simulink model "pose_ctrl_R2017a"  (R2017a)
settings: Solver=FixedStepAuto  StartTime=0.0  StopTime=20  FixedStep=0.0005  RelTol=1e-3
InitFcn:
  | Parameter
values from neighbouring files (symbols this model uses):
  alpha = pi/180 * 13.6    (= 0.237364778271)    [IdealParameter.m]    (also in ParLuk11.m = deg2rad(13.6); Parameter.m = [-alpha_i;alpha_i;-alpha_i;alpha_i;-alpha_i;alpha_i]; ParameterIdeal.m = [-alpha_i;alpha_i;-alpha_i;alpha_i;-alpha_i;alpha_i]; ParameterVIVE.m = [alpha_i;-alpha_i;alpha_i;-alpha_i;alpha_i;-alpha_i])
  alpha_0 = alpha    (= 0.237364778271)    [IdealParameter.m]    (also in Parameter.m = alpha; ParameterIdeal.m = alpha*1.01; ParameterVIVE.m = alpha*1.01; ParameterVO.m = alpha*1.01)
  angular_noise = 0    [IdealParameter.m]    (also in Parameter.m = 0.5; ParameterIdeal.m; ParameterVIVE.m; ParameterVO.m)
  b = 1.1e-06    [IdealParameter.m]    (also in ParLuk11.m = 1.14e-07; Parameter.m = 8.944e-07; ParameterIdeal.m; ParameterVIVE.m)
  b_0 = b*1.15    (= 1.265e-06)    [IdealParameter.m]    (also in Parameter.m = 8.944e-07; ParameterIdeal.m; ParameterVIVE.m; ParameterVO.m)
  beta = 0    [IdealParameter.m]    (also in ParLuk11.m; Parameter.m = [beta_i; beta_i; beta_i; beta_i; beta_i; beta_i]; ParameterIdeal.m = [beta_i; beta_i; beta_i; beta_i; beta_i; beta_i]; ParameterVIVE.m = [beta_i; beta_i; beta_i; beta_i; beta_i; beta_i])
  beta_0 = beta    (= 0)    [IdealParameter.m]    (also in Parameter.m = beta; ParameterIdeal.m = beta*0.99; ParameterVIVE.m = beta*0.99; ParameterVO.m = beta*0.99)
  eta = 1    [Controllability.m]    (also in IdealParameter.m = 75; Parameter.m = 2; ParameterIdeal.m = 40; ParameterVIVE.m = 10)
  eta_rot = 50    [IdealParameter.m]    (also in Parameter.m = 2; ParameterIdeal.m = 20; ParameterVIVE.m = 5; ParameterVO.m = 2)
  g = 9.81    [IdealParameter.m]    (also in ParLuk11.m; Parameter.m; ParameterIdeal.m; ParameterVIVE.m)
  g_0 = g*0.99    (= 9.7119)    [IdealParameter.m]    (also in Parameter.m = 9.81; ParameterIdeal.m = 9.81; ParameterVIVE.m = 9.81; ParameterVO.m = 9.81)
  IB = [Ixx 0 0; 0 Iyy 0; 0 0 Izz]    [IdealParameter.m]    (also in ParLuk11.m; Parameter.m; ParameterIdeal.m; ParameterVIVE.m)
  IB_0 = IB*1.07    [IdealParameter.m]    (also in Parameter.m = IB; ParameterIdeal.m; ParameterVIVE.m; ParameterVO.m)
  k = 5.6e-05    [IdealParameter.m]    (also in ParLuk11.m = 2.98e-06; Parameter.m = 4.472e-05; ParameterIdeal.m; ParameterVIVE.m = 5.13e-05)
  K_0 = Ts/(T_rotor_0+Ts)    (= 0.0384615384615)    [IdealParameter.m]    (also in Parameter.m = 0.230769230769; ParameterIdeal.m; ParameterVIVE.m = 0.0350877192982; ParameterVO.m = 0.214285714286)
  k_0 = k*1.16    (= 6.496e-05)    [IdealParameter.m]    (also in Parameter.m = 4.472e-05; ParameterIdeal.m; ParameterVIVE.m = 5.9508e-05; ParameterVO.m)
  K_P_1 = 15*eye(3)    [IdealParameter.m]    (also in Parameter.m = 2*eye(3); ParameterIdeal.m; ParameterVIVE.m = 10*eye(3); ParameterVO.m = 2*eye(3))
  K_P_2 = 50*eye(3)    [IdealParameter.m]    (also in Parameter.m = 4*eye(3); ParameterIdeal.m; ParameterVIVE.m = 10*eye(3); ParameterVO.m = 4*eye(3))
  K_P_3 = 60*eye(3)    [IdealParameter.m]    (also in Parameter.m = 6*eye(3); ParameterIdeal.m; ParameterVIVE.m = 10*eye(3); ParameterVO.m = 6*eye(3))
  K_P_D = 30*eye(3)    [IdealParameter.m]    (also in ParLuk11.m = 10*eye(3); Parameter.m = 5*eye(3); ParameterIdeal.m; ParameterVIVE.m = 15*eye(3))
  K_P_I = 100*eye(3)    [IdealParameter.m]    (also in ParLuk11.m = 10*eye(3); Parameter.m = 10*eye(3); ParameterIdeal.m = 80*eye(3); ParameterVIVE.m)
  K_P_P = 100*eye(3)    [IdealParameter.m]    (also in ParLuk11.m = 20*eye(3); Parameter.m = 10*eye(3); ParameterIdeal.m = 130*eye(3); ParameterVIVE.m)
  K_R_1 = 40*eye(3)    [IdealParameter.m]    (also in Parameter.m = 2*eye(3); ParameterIdeal.m; ParameterVIVE.m = 10*eye(3); ParameterVO.m = 2*eye(3))
  K_R_2 = 100*eye(3)    [IdealParameter.m]    (also in Parameter.m = 4*eye(3); ParameterIdeal.m; ParameterVIVE.m = 10*eye(3); ParameterVO.m = 4*eye(3))
  K_R_3 = 50*eye(4)    [IdealParameter.m]    (also in Parameter.m = 6*eye(4); ParameterIdeal.m; ParameterVIVE.m = 10*eye(4); ParameterVO.m = 6*eye(4))
  K_R_D = 30*eye(3)    [IdealParameter.m]    (also in ParLuk11.m = 10*eye(3); Parameter.m = 5*eye(3); ParameterIdeal.m; ParameterVIVE.m = 15*eye(3))
  K_R_I = 100*eye(3)    [IdealParameter.m]    (also in ParLuk11.m = 10*eye(3); Parameter.m = 10*eye(3); ParameterIdeal.m = 80*eye(3); ParameterVIVE.m)
  K_R_P = 100*eye(3)    [IdealParameter.m]    (also in ParLuk11.m = 20*eye(3); Parameter.m = 10*eye(3); ParameterIdeal.m = 130*eye(3); ParameterVIVE.m)
  L = 0.4    [IdealParameter.m]    (also in ParLuk11.m = 1; Parameter.m; ParameterIdeal.m; ParameterVIVE.m = 0.6)
  L_0 = L*1.02    (= 0.408)    [IdealParameter.m]    (also in Parameter.m = 0.4; ParameterIdeal.m; ParameterVIVE.m = 0.612; ParameterVO.m)
  lambda = 10    [IdealParameter.m]    (also in Parameter.m = 3; ParameterIdeal.m = 5; ParameterVIVE.m = 5; ParameterVO.m = 3)
  lambda_rot = 10    [IdealParameter.m]    (also in Parameter.m = 3; ParameterIdeal.m; ParameterVIVE.m = 5; ParameterVO.m = 3)
  M = 50    [IdealParameter.m]    (also in Parameter.m = 6; ParameterIdeal.m = 100; ParameterVIVE.m = 5; ParameterVO.m = 6)
  m = 1    [Controllability.m]    (also in IdealParameter.m = 2.5; ParLuk11.m = 0.6; Parameter.m = 4.85; ParameterIdeal.m = 4.85)
  m_0 = m*1.03    (= 2.575)    [IdealParameter.m]    (also in Parameter.m = 4.85; ParameterIdeal.m = 4.9955; ParameterVIVE.m = 4.52994; ParameterVO.m = 4.9955)
  M_rot = 50    [IdealParameter.m]    (also in Parameter.m = 6; ParameterIdeal.m = 15; ParameterVIVE.m = 1; ParameterVO.m = 6)
  omega_noise = 0    [IdealParameter.m]    (also in Parameter.m = sqrt(2)*angular_noise/Ts * pi/180; ParameterIdeal.m; ParameterVIVE.m; ParameterVO.m)
  p_noise = 0    [IdealParameter.m]    (also in Parameter.m = 0.001; ParameterIdeal.m; ParameterVIVE.m; ParameterVO.m)
  T_delay = 0    [IdealParameter.m]    (also in Parameter.m = 0.1; ParameterIdeal.m; ParameterVIVE.m = 0.04; ParameterVO.m = 0.1)
  T_rotor = 0.1    [IdealParameter.m]    (also in Parameter.m; ParameterIdeal.m; ParameterVIVE.m; ParameterVO.m)
  Ts = 1/250    (= 0.004)    [IdealParameter.m]    (also in Parameter.m = 0.03; ParameterIdeal.m; ParameterVIVE.m; ParameterVO.m = 0.03)
  v_noise = 0    [IdealParameter.m]    (also in Parameter.m = sqrt(2)*p_noise/Ts; ParameterIdeal.m; ParameterVIVE.m; ParameterVO.m)
  z_p_0 = T_rotor_0/(T_rotor_0+Ts)    (= 0.961538461538)    [IdealParameter.m]    (also in Parameter.m = 0.769230769231; ParameterIdeal.m; ParameterVIVE.m = 0.964912280702; ParameterVO.m = 0.785714285714)
undefined symbols (not defined in the file or in its folder): DiscIntNeverNeededParam
libraries: simulink x7, vrlib x3, dspmtrx3 x1
(part 1 of 2)
settings Model: Creator=jan  LastModifiedBy=chao

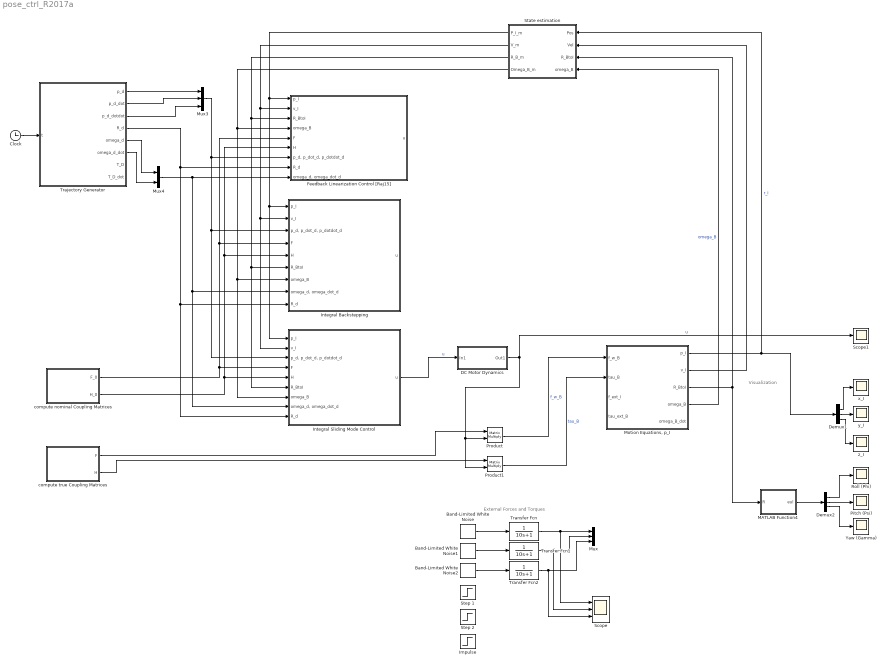
== system pose_ctrl_R2017a ==
  note: External Forces and Torques
  note: Visualization
  Band-Limited White Noise : simulink/Sources/Band-Limited White Noise  Cov=10  Ts=0.1  seed=[28341]  VectorParams1D=off
  Band-Limited White Noise1 : simulink/Sources/Band-Limited White Noise  Cov=10  Ts=0.1  seed=[23342]  VectorParams1D=off
  Band-Limited White Noise2 : simulink/Sources/Band-Limited White Noise  Cov=10  Ts=0.1  seed=[23441]  VectorParams1D=off
  Clock : Clock
  "DC Motor Dynamics " : Subsystem  TreatAsAtomicUnit=on
  Demux1 : Demux  Outputs=3
  Demux2 : Demux  Outputs=3
  Feedback Linearization Control [Raj15] : Subsystem
  Impulse : Step  Time=0.1  Before=[6,0,6]'  After=[0,0,0]'  SampleTime=0  VectorParams1D=off
  Integral Backstepping : Subsystem
  Integral Sliding Mode Control : Subsystem
  MATLAB Function4 : MATLAB Function  TreatAsAtomicUnit=on
  "Motion Equations, p_I" : Subsystem
  Mux : Mux  Inputs=3
  Mux3 : Mux  Inputs=3
  Mux4 : Mux  Inputs=2
  Pitch (Psi) : Scope
  Product : Product  Multiplication=Matrix(*)
  Product1 : Product  Multiplication=Matrix(*)
  Roll (Phi) : Scope
  Scope : Scope  NumInputPorts=3
  Scope1 : Scope
  State estimation : Subsystem
  Step 1 : Step  Before=[0;0;0]  After=[10;1;1]  SampleTime=0  VectorParams1D=off
  Step 2 : Step  Before=[0;0;0]  After=[5;1;1]  SampleTime=0  VectorParams1D=off
  Trajectory Generator : MATLAB Function  TreatAsAtomicUnit=on
  Transfer Fcn : TransferFcn  Denominator=[10 1]
  Transfer Fcn1 : TransferFcn  Denominator=[10 1]
  Transfer Fcn2 : TransferFcn  Denominator=[10 1]
  Yaw (Gamma) : Scope
  compute nominal Coupling Matrices : Subsystem
  compute true Coupling Matrices : Subsystem
  x_I : Scope
  y_I : Scope
  z_I : Scope
  wires:
  Demux2/2 -> Pitch (Psi)/1
  Demux1/3 -> z_I/1
  Demux1/1 -> x_I/1
  "DC Motor Dynamics "/1(Out1) -> Product1/2, Product/2, Scope1/1  "u"
  Demux1/2 -> y_I/1
  Demux2/1 -> Roll (Phi)/1
  compute nominal Coupling Matrices/1(F_0) -> Integral Backstepping/4(F), Feedback Linearization Control [Raj15]/5(F), Integral Sliding Mode Control/4(F)
  Product/1 -> "Motion Equations, p_I"/1("f_w_B ")  "f_w_B"
  compute nominal Coupling Matrices/2("H_0 ") -> Integral Backstepping/5(H), Feedback Linearization Control [Raj15]/6(H), Integral Sliding Mode Control/5(H)
  Product1/1 -> "Motion Equations, p_I"/2(tau_B)  "tau_B"
  Clock/1 -> Trajectory Generator/1(t)
  Trajectory Generator/3(p_d_dotdot) -> Mux3/3
  Trajectory Generator/2(p_d_dot) -> Mux3/2
  Trajectory Generator/1(p_d) -> Mux3/1
  Trajectory Generator/6(omega_d_dot) -> Mux4/2
  Band-Limited White Noise/1 -> Transfer Fcn/1
  Transfer Fcn/1 -> Scope/1, Mux/1
  Transfer Fcn2/1 -> Scope/3, Mux/3
  Band-Limited White Noise1/1 -> Transfer Fcn1/1
  Band-Limited White Noise2/1 -> Transfer Fcn2/1
  Transfer Fcn1/1 -> Scope/2, Mux/2
  Mux3/1 -> Integral Sliding Mode Control/3("p_d, p_dot_d, p_dotdot_d"), Integral Backstepping/3("p_d, p_dot_d, p_dotdot_d"), Feedback Linearization Control [Raj15]/7("p_d, p_dot_d, p_dotdot_d")
  Trajectory Generator/4(R_d) -> Integral Sliding Mode Control/9(R_d), Integral Backstepping/9(R_d), Feedback Linearization Control [Raj15]/8(R_d)
  Trajectory Generator/5(omega_d) -> Mux4/1
  Mux4/1 -> Integral Sliding Mode Control/8("omega_d, omega_dot_d"), Integral Backstepping/8("omega_d, omega_dot_d"), Feedback Linearization Control [Raj15]/9("omega_d, omega_dot_d")
  compute true Coupling Matrices/1(F) -> Product/1
  compute true Coupling Matrices/2(H) -> Product1/1
  "Motion Equations, p_I"/1(p_I) -> Demux1/1, State estimation/1(Pos)  "r_I"
  "Motion Equations, p_I"/3(R_BtoI) -> State estimation/3(R_BtoI), MATLAB Function4/1(R)
  Demux2/3 -> Yaw (Gamma)/1
  MATLAB Function4/1(eul) -> Demux2/1
  Integral Sliding Mode Control/1(u) -> "DC Motor Dynamics "/1(In1)  "u"
  State estimation/3(R_B_m) -> Integral Sliding Mode Control/6(R_BtoI), Integral Backstepping/6(R_BtoI), Feedback Linearization Control [Raj15]/3("R_BtoI ")
  State estimation/2(V_m) -> Integral Sliding Mode Control/2(v_I), Integral Backstepping/2(v_I), Feedback Linearization Control [Raj15]/2(v_I)
  State estimation/1(P_I_m) -> Integral Sliding Mode Control/1(p_I), Integral Backstepping/1(p_I), Feedback Linearization Control [Raj15]/1("p_I ")
  State estimation/4(Omega_B_m) -> Integral Sliding Mode Control/7(omega_B), Integral Backstepping/7(omega_B), Feedback Linearization Control [Raj15]/4(omega_B)
  "Motion Equations, p_I"/2(v_I) -> State estimation/2(Vel)
  "Motion Equations, p_I"/4(omega_B) -> State estimation/4(omega_B)  "omega_B"

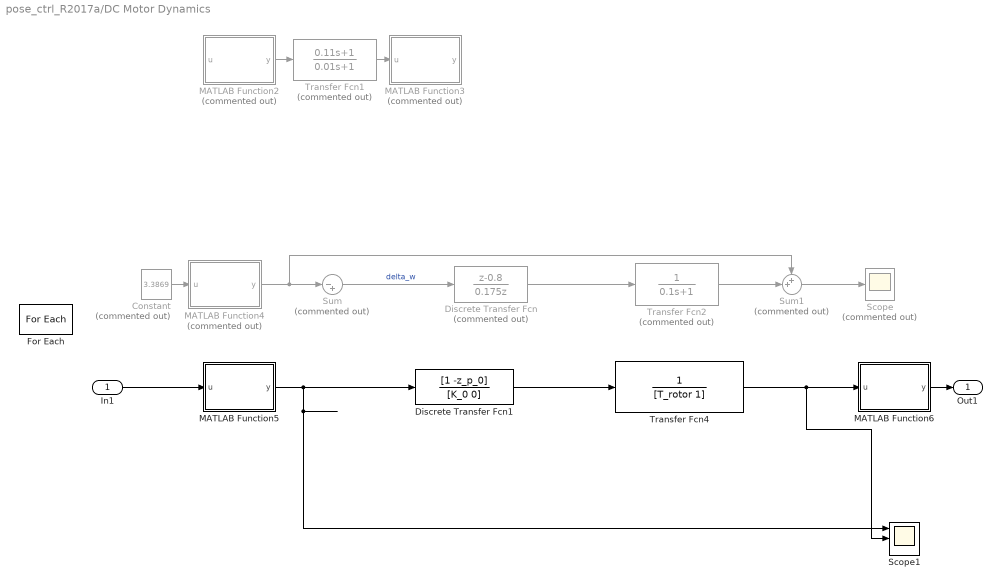
== system pose_ctrl_R2017a/DC Motor Dynamics  ==
  In1 : Inport  Partition=on  PartitionDimension=1  PartitionWidth=1
  Constant : Constant  Commented=on  Value=3.3869
  Discrete Transfer Fcn : DiscreteTransferFcn  Commented=on  Numerator=[1 -0.8]  Denominator=[0.175 0]  SampleTime=Ts
  Discrete Transfer Fcn1 : DiscreteTransferFcn  Numerator=[1 -z_p_0]  Denominator=[K_0 0]  SampleTime=Ts
  For Each : ForEach  DisableCoverage=on  IndexMode=One-based
  MATLAB Function2 : MATLAB Function  Commented=on  TreatAsAtomicUnit=on
  MATLAB Function3 : MATLAB Function  Commented=on  TreatAsAtomicUnit=on
  MATLAB Function4 : MATLAB Function  Commented=on  TreatAsAtomicUnit=on
  MATLAB Function5 : MATLAB Function  TreatAsAtomicUnit=on  SystemSampleTime=Ts
  MATLAB Function6 : MATLAB Function  TreatAsAtomicUnit=on
  Scope : Scope  Commented=on
  Scope1 : Scope  NumInputPorts=3
  Sum : Sum  Commented=on  Inputs=|-+
  Sum1 : Sum  Commented=on  Inputs=++|
  Transfer Fcn1 : TransferFcn  Commented=on  Numerator=[0.11 1]  Denominator=[0.01 1]
  Transfer Fcn2 : TransferFcn  Commented=on  Denominator=[0.1 1]
  Transfer Fcn4 : TransferFcn  Denominator=[T_rotor 1]
  Out1 : Outport  ConcatenationDimension=1
  wires:
  Transfer Fcn1/1 -> MATLAB Function3/1(u)
  MATLAB Function2/1(y) -> Transfer Fcn1/1
  Constant/1 -> MATLAB Function4/1(u)
  MATLAB Function4/1(y) -> Sum1/1, Sum/1
  Sum/1 -> Discrete Transfer Fcn/1  "delta_w"
  In1/1 -> MATLAB Function5/1(u)
  MATLAB Function5/1(y) -> Discrete Transfer Fcn1/1, Scope1/1
  Discrete Transfer Fcn/1 -> Transfer Fcn2/1
  Transfer Fcn2/1 -> Sum1/2
  MATLAB Function6/1(y) -> Out1/1
  Sum1/1 -> Scope/1
  Discrete Transfer Fcn1/1 -> Transfer Fcn4/1
  Transfer Fcn4/1 -> Scope1/2, MATLAB Function6/1(u)

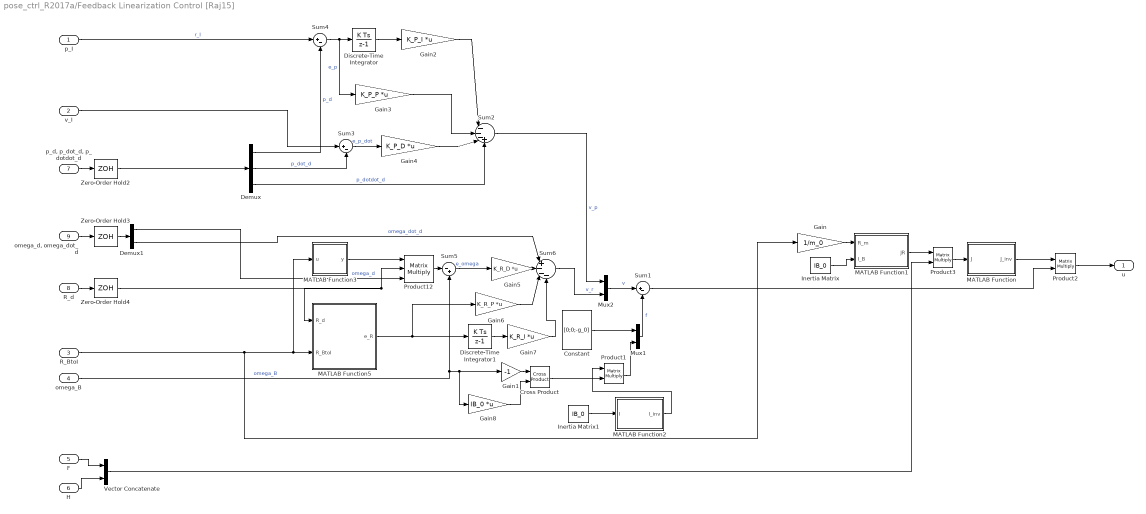
== system pose_ctrl_R2017a/Feedback Linearization Control [Raj15] ==
  "p_I " : Inport
  v_I : Inport  Port=2
  "R_BtoI " : Inport  Port=3
  omega_B : Inport  Port=4
  F : Inport  Port=5
  H : Inport  Port=6
  "p_d, p_dot_d, p_dotdot_d" : Inport  Port=7
  R_d : Inport  Port=8
  "omega_d, omega_dot_d" : Inport  Port=9
  Constant : Constant  Value=[0;0;-g_0]  VectorParams1D=off
  Cross Product : vrlib/Utilities/Cross Product
      settings: SourceProductBaseCode=VR
  Demux : Demux  Outputs=3
  Demux1 : Demux  Outputs=2
  Discrete-Time Integrator : DiscreteIntegrator  InitialCondition=[0;0;0]  InitialConditionSetting=State (most efficient)  SampleTime=Ts  ICPrevOutput=DiscIntNeverNeededParam  ICPrevScaledInput=DiscIntNeverNeededParam
  Discrete-Time Integrator1 : DiscreteIntegrator  InitialCondition=[0;0;0]  InitialConditionSetting=State (most efficient)  SampleTime=Ts  ICPrevOutput=DiscIntNeverNeededParam  ICPrevScaledInput=DiscIntNeverNeededParam
  Gain : Gain  Gain=1/m_0
  Gain1 : Gain  Gain=-1
  Gain2 : Gain  Gain=K_P_I  Multiplication=Matrix(K*u)
  Gain3 : Gain  Gain=K_P_P  Multiplication=Matrix(K*u)
  Gain4 : Gain  Gain=K_P_D  Multiplication=Matrix(K*u)
  Gain5 : Gain  Gain=K_R_D  Multiplication=Matrix(K*u)
  Gain6 : Gain  Gain=K_R_P  Multiplication=Matrix(K*u)
  Gain7 : Gain  Gain=K_R_I  Multiplication=Matrix(K*u)
  Gain8 : Gain  Gain=IB_0  Multiplication=Matrix(K*u)
  Inertia Matrix : Constant  Value=IB_0  VectorParams1D=off
  Inertia Matrix1 : Constant  Value=IB_0  VectorParams1D=off
  MATLAB Function : MATLAB Function  TreatAsAtomicUnit=on
  MATLAB Function1 : MATLAB Function  TreatAsAtomicUnit=on
  MATLAB Function2 : MATLAB Function  TreatAsAtomicUnit=on
  MATLAB Function3 : MATLAB Function  TreatAsAtomicUnit=on
  MATLAB Function5 : MATLAB Function  TreatAsAtomicUnit=on
  Mux1 : Mux  Inputs=2
  Mux2 : Mux  Inputs=2
  Product1 : Product  Multiplication=Matrix(*)
  Product12 : Product  Inputs=***  Multiplication=Matrix(*)
  Product2 : Product  Multiplication=Matrix(*)
  Product3 : Product  Multiplication=Matrix(*)
  Sum1 : Sum  Inputs=|+-
  Sum2 : Sum  Inputs=|---+
  Sum3 : Sum  Inputs=|+-
  Sum4 : Sum  Inputs=|+-
  Sum5 : Sum  Inputs=|-+
  Sum6 : Sum  Inputs=|+---
  Vector Concatenate : Concatenate  Mode=Multidimensional array
  Zero-Order Hold2 : ZeroOrderHold  SampleTime=Ts
  Zero-Order Hold3 : ZeroOrderHold  SampleTime=Ts
  Zero-Order Hold4 : ZeroOrderHold  SampleTime=Ts
  u : Outport
  wires:
  Demux/1 -> Sum4/2  "p_d"
  Sum2/1 -> Mux2/1  "v_p"
  Demux/3 -> Sum2/4  "p_dotdot_d"
  "p_I "/1 -> Sum4/1  "r_I"
  Gain3/1 -> Sum2/2
  Discrete-Time Integrator/1 -> Gain2/1
  Sum4/1 -> Discrete-Time Integrator/1, Gain3/1  "e_p"
  Demux/2 -> Sum3/2  "p_dot_d"
  Gain2/1 -> Sum2/1
  Sum3/1 -> Gain4/1  "e_p_dot"
  "p_d, p_dot_d, p_dotdot_d"/1 -> Zero-Order Hold2/1
  Gain4/1 -> Sum2/3
  R_d/1 -> Zero-Order Hold4/1
  Gain5/1 -> Sum6/2
  Gain6/1 -> Sum6/3
  Mux1/1 -> Sum1/2  "f"
  Vector Concatenate/1 -> Product3/2
  Discrete-Time Integrator1/1 -> Gain7/1
  Product3/1 -> MATLAB Function/1(J)
  omega_B/1 -> Gain8/1, Gain1/1, Sum5/2  "omega_B"
  Constant/1 -> Mux1/1
  Gain/1 -> MATLAB Function1/1(R_m)
  MATLAB Function/1(J_inv) -> Product2/1
  Sum1/1 -> Product2/2
  Gain7/1 -> Sum6/4
  MATLAB Function1/1(JR) -> Product3/1
  Product12/1 -> Sum5/1
  Gain1/1 -> Cross Product/1
  Mux2/1 -> Sum1/1  "v"
  MATLAB Function5/1(e_R) -> Discrete-Time Integrator1/1, Gain6/1
  Inertia Matrix/1 -> MATLAB Function1/2(I_B)
  Sum6/1 -> Mux2/2  "v_r"
  Gain8/1 -> Cross Product/2
  Demux1/2 -> Sum6/1  "omega_dot_d"
  MATLAB Function3/1(y) -> Product12/1
  Demux1/1 -> Product12/3  "omega_d"
  Cross Product/1 -> Product1/2
  Sum5/1 -> Gain5/1  "e_omega"
  F/1 -> Vector Concatenate/1
  H/1 -> Vector Concatenate/2
  "omega_d, omega_dot_d"/1 -> Zero-Order Hold3/1
  Product2/1 -> u/1
  Product1/1 -> Mux1/2
  Inertia Matrix1/1 -> MATLAB Function2/1(I)
  MATLAB Function2/1(I_inv) -> Product1/1
  v_I/1 -> Sum3/1
  Zero-Order Hold2/1 -> Demux/1
  Zero-Order Hold3/1 -> Demux1/1
  Zero-Order Hold4/1 -> Product12/2, MATLAB Function5/1(R_d)
  "R_BtoI "/1 -> Gain/1, MATLAB Function5/2(R_BtoI), MATLAB Function3/1(u)

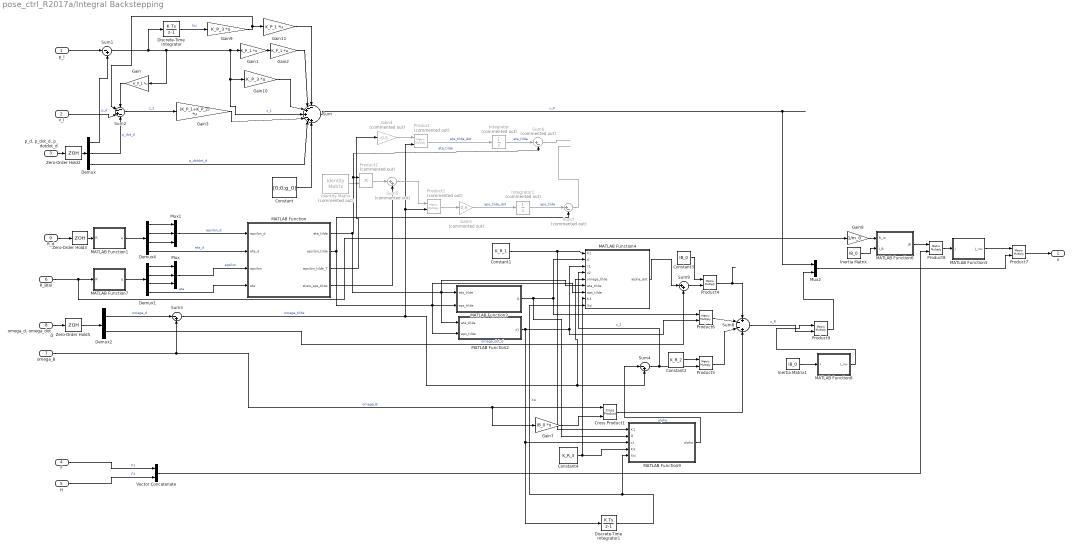
== system pose_ctrl_R2017a/Integral Backstepping ==
  p_I : Inport
  v_I : Inport  Port=2
  "p_d, p_dot_d, p_dotdot_d" : Inport  Port=3
  F : Inport  Port=4
  H : Inport  Port=5
  R_BtoI : Inport  Port=6
  omega_B : Inport  Port=7
  "omega_d, omega_dot_d" : Inport  Port=8
  R_d : Inport  Port=9
  Constant : Constant  Value=[0;0;g_0]  VectorParams1D=off
  Constant1 : Constant  Value=K_R_1  VectorParams1D=off
  Constant2 : Constant  Value=K_R_2  VectorParams1D=off
  Constant3 : Constant  Value=IB_0  VectorParams1D=off
  Constant4 : Constant  Value=K_R_3  VectorParams1D=off
  Cross Product1 : vrlib/Utilities/Cross Product
      settings: SourceProductBaseCode=VR
  Demux : Demux  Outputs=3
  Demux1 : Demux
  Demux2 : Demux  Outputs=2
  Demux4 : Demux
  Discrete-Time Integrator : DiscreteIntegrator  InitialCondition=[0;0;0]  InitialConditionSetting=State (most efficient)  SampleTime=Ts  ICPrevOutput=DiscIntNeverNeededParam  ICPrevScaledInput=DiscIntNeverNeededParam
  Discrete-Time Integrator1 : DiscreteIntegrator  InitialCondition=[0;0;0;0]  InitialConditionSetting=State (most efficient)  SampleTime=Ts  ICPrevOutput=DiscIntNeverNeededParam  ICPrevScaledInput=DiscIntNeverNeededParam
  Gain{,1..2,11} (4 alike) : Gain  Gain=K_P_1  Multiplication=Matrix(K*u)
  Gain10 : Gain  Gain=K_P_3  Multiplication=Matrix(K*u)
  Gain3 : Gain  Gain=(K_P_1+K_P_2)  Multiplication=Matrix(K*u)
  Gain4 : Gain  Commented=on  Gain=-0.5
  Gain5 : Gain  Commented=on  Gain=0.5
  Gain7 : Gain  Gain=IB_0  Multiplication=Matrix(K*u)
  Gain8 : Gain  Gain=1/m_0
  Gain9 : Gain  Gain=K_P_3  Multiplication=Matrix(K*u)
  Identity Matrix : dspmtrx3/Identity Matrix  Commented=on  Inherit=off  N=3  Ts=inf  dataType=double  isSigned=on  wordLen=16  udDataType=sfix(16)  fracBitsMode=Best precision  numFracBits=15  OutDataTypeStr=double  LastOutDataTypeStr=double
      settings: SourceProductName=DSP System Toolbox
  Inertia Matrix : Constant  Value=IB_0  VectorParams1D=off
  Inertia Matrix1 : Constant  Value=IB_0  VectorParams1D=off
  Integrator : Integrator  Commented=on  InitialCondition=1
  Integrator1 : Integrator  Commented=on  InitialCondition=[0;0;0]
  MATLAB Function : MATLAB Function  TreatAsAtomicUnit=on
  MATLAB Function1 : MATLAB Function  TreatAsAtomicUnit=on
  MATLAB Function2 : MATLAB Function  TreatAsAtomicUnit=on
  MATLAB Function3 : MATLAB Function  TreatAsAtomicUnit=on
  MATLAB Function4 : MATLAB Function  TreatAsAtomicUnit=on
  MATLAB Function5 : MATLAB Function  TreatAsAtomicUnit=on
  MATLAB Function6 : MATLAB Function  TreatAsAtomicUnit=on
  MATLAB Function7 : MATLAB Function  TreatAsAtomicUnit=on
  MATLAB Function8 : MATLAB Function  TreatAsAtomicUnit=on
  MATLAB Function9 : MATLAB Function  TreatAsAtomicUnit=on
  Mux : Mux  Inputs=3
  Mux1 : Mux  Inputs=3
  Mux2 : Mux  Inputs=2
  Product : Product  Commented=on  Multiplication=Matrix(*)
  Product1 : Product  Commented=on  Multiplication=Matrix(*)
  Product2 : Product  Commented=on
  Product{4..9} (6 alike) : Product  Multiplication=Matrix(*)
  Sum : Sum  Inputs=--++-++
  Sum1 : Sum  Inputs=|-+
  Sum2 : Sum  Inputs=--+-
  Sum3 : Sum  Inputs=|-+
  Sum4 : Sum  Inputs=|-+
  Sum5 : Sum  Commented=on  Inputs=|++
  Sum6 : Sum  Commented=on  Inputs=|+-
  Sum7 : Sum  Commented=on  Inputs=|+-
  Sum8 : Sum  Inputs=+--+
  Sum9 : Sum  Inputs=|++
  Vector Concatenate : Concatenate  Mode=Multidimensional array
  Zero-Order Hold2 : ZeroOrderHold  SampleTime=Ts
  Zero-Order Hold3 : ZeroOrderHold  SampleTime=Ts
  Zero-Order Hold5 : ZeroOrderHold  SampleTime=Ts
  u : Outport
  wires:
  F/1 -> Vector Concatenate/1  "F1"
  H/1 -> Vector Concatenate/2  "F2"
  Sum2/1 -> Gain3/1  "z_2"
  Sum1/1 -> Discrete-Time Integrator/1, Sum/4, Gain10/1, Gain1/1, Gain/1  "z_1"
  Gain/1 -> Sum2/1
  Demux/2 -> Sum2/4  "p_dot_d"
  Demux/3 -> Sum/6  "p_dotdot_d"
  "p_d, p_dot_d, p_dotdot_d"/1 -> Zero-Order Hold2/1
  Demux/1 -> Sum1/2  "p_d"
  Sum/1 -> Mux2/1  "u_P"
  Gain1/1 -> Gain2/1
  Gain2/1 -> Sum/2
  Constant/1 -> Sum/7
  Gain3/1 -> Sum/5
  MATLAB Function7/1(q) -> Demux1/1
  Demux1/1 -> Mux/1
  Demux1/2 -> Mux/2
  Demux1/3 -> Mux/3
  Demux1/4 -> MATLAB Function/4(eta)  "eta"
  Mux/1 -> MATLAB Function/3(epsilon)  "epsilon"
  Demux2/2 -> Sum9/2  "omega_dot_d"
  "omega_d, omega_dot_d"/1 -> Zero-Order Hold5/1
  Demux2/1 -> Sum3/1  "omega_d"
  Demux4/3 -> Mux1/3
  MATLAB Function1/1(q) -> Demux4/1
  Demux4/4 -> MATLAB Function/2(eta_d)  "eta_d"
  Demux4/1 -> Mux1/1
  Demux4/2 -> Mux1/2
  Mux1/1 -> MATLAB Function/1(epsilon_d)  "epsilon_d"
  Zero-Order Hold3/1 -> MATLAB Function1/1(R)
  Sum3/1 -> MATLAB Function4/5(omega_tilde), Sum4/2, Product/2, Product1/2  "omega_tilde"
  Gain4/1 -> Product/1
  Product/1 -> Integrator/1  "eta_tilde_dot"
  Integrator/1 -> Sum6/1  "eta_tilde"
  Product1/1 -> Gain5/1
  Identity Matrix/1 -> Product2/2
  MATLAB Function/1(eta_tilde) -> MATLAB Function4/6(eta_tilde), MATLAB Function2/1(eta_tilde), MATLAB Function3/1(eta_tilde), Sum6/2, Product2/1  "eta_tilde"
  Product2/1 -> Sum5/1
  MATLAB Function/4(skew_eps_tilde) -> Sum5/2
  Sum5/1 -> Product1/1
  Gain5/1 -> Integrator1/1  "eps_tilde_dot"
  Integrator1/1 -> Sum7/1  "eps_tilde"
  MATLAB Function/2(epsilon_tilde) -> MATLAB Function4/7(eps_tilde), MATLAB Function2/2(eps_tilde), MATLAB Function3/2(eps_tilde), Sum7/2
  Sum7/1 -> ?
  Sum6/1 -> ?
  MATLAB Function/3(epsilon_tilde_T) -> Gain4/1
  Constant1/1 -> MATLAB Function9/1(K1), MATLAB Function4/1(K1)
  MATLAB Function3/1(G) -> MATLAB Function9/2(G), Product6/1, MATLAB Function4/2(G)
  MATLAB Function2/1(z1) -> Product6/2, MATLAB Function4/3(z1), MATLAB Function9/3(z1), Discrete-Time Integrator1/1
  MATLAB Function9/1(alpha) -> Sum4/1  "alpha"
  Sum4/1 -> Product5/2, MATLAB Function4/4(z2)  "z_2"
  MATLAB Function4/1(alpha_dot) -> Sum9/1
  Sum9/1 -> Product4/2
  Constant3/1 -> Product4/1
  Product4/1 -> Sum8/1
  Gain7/1 -> Cross Product1/2
  omega_B/1 -> Gain7/1, Cross Product1/1, Sum3/2  "omega_B"
  Cross Product1/1 -> Sum8/4
  Product5/1 -> Sum8/3
  Constant2/1 -> Product5/1
  Product6/1 -> Sum8/2
  Sum8/1 -> Product9/2  "u_R"
  MATLAB Function5/1(J_inv) -> Product7/1
  Inertia Matrix/1 -> MATLAB Function6/2(I_B)
  Gain8/1 -> MATLAB Function6/1(R_m)
  Vector Concatenate/1 -> Product8/2
  Product7/1 -> u/1
  MATLAB Function6/1(JR) -> Product8/1
  Product8/1 -> MATLAB Function5/1(J)
  R_BtoI/1 -> Gain8/1, MATLAB Function7/1(R)
  Mux2/1 -> Product7/2
  Inertia Matrix1/1 -> MATLAB Function8/1(I)
  MATLAB Function8/1(I_inv) -> Product9/1
  Product9/1 -> Mux2/2
  Discrete-Time Integrator/1 -> Gain9/1  "Xsi"
  Gain9/1 -> Gain11/1, Sum2/2
  Gain10/1 -> Sum/3
  Gain11/1 -> Sum/1
  Discrete-Time Integrator1/1 -> MATLAB Function4/9(Xsi), MATLAB Function9/5(Xsi)  "Xsi"
  Constant4/1 -> MATLAB Function9/4(K3), MATLAB Function4/8(K3)
  p_I/1 -> Sum1/1
  v_I/1 -> Sum2/3
  Zero-Order Hold2/1 -> Demux/1
  R_d/1 -> Zero-Order Hold3/1
  Zero-Order Hold5/1 -> Demux2/1

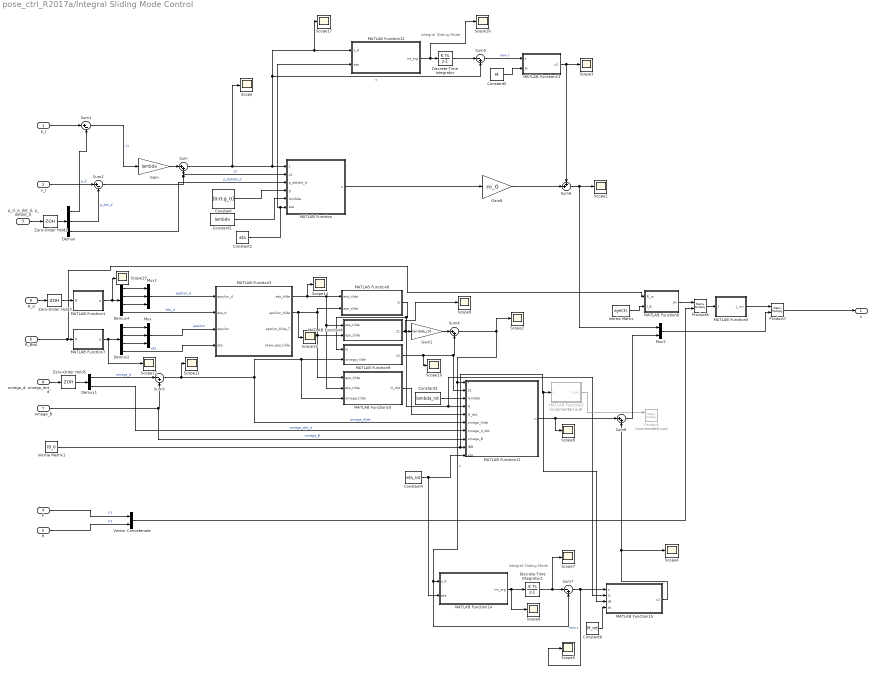
== system pose_ctrl_R2017a/Integral Sliding Mode Control ==
  note: Integral Sliding Mode
  note: Integral Sliding Mode
  p_I : Inport
  v_I : Inport  Port=2
  "p_d, p_dot_d, p_dotdot_d" : Inport  Port=3
  F : Inport  Port=4
  H : Inport  Port=5
  R_BtoI : Inport  Port=6
  omega_B : Inport  Port=7
  "omega_d, omega_dot_d" : Inport  Port=8
  R_d : Inport  Port=9
  Constant : Constant  Value=[0;0;g_0]  VectorParams1D=off
  Constant1 : Constant  Value=lambda
  Constant2 : Constant  Value=eta
  Constant3 : Constant  Value=lambda_rot
  Constant4 : Constant  Value=eta_rot
  Constant5 : Constant  Value=M
  Constant6 : Constant  Value=M_rot
  Demux : Demux  Outputs=3
  Demux1 : Demux  Outputs=2
  Demux2 : Demux
  Demux4 : Demux
  Discrete-Time Integrator : DiscreteIntegrator  InitialCondition=[0;0;0]  InitialConditionSetting=State (most efficient)  SampleTime=Ts  ICPrevOutput=DiscIntNeverNeededParam  ICPrevScaledInput=DiscIntNeverNeededParam
  Discrete-Time Integrator1 : DiscreteIntegrator  InitialCondition=[0;0;0;0]  InitialConditionSetting=State (most efficient)  SampleTime=Ts  ICPrevOutput=DiscIntNeverNeededParam  ICPrevScaledInput=DiscIntNeverNeededParam
  Gain : Gain  Gain=lambda
  Gain1 : Gain  Gain=lambda_rot
  Gain8 : Gain  Gain=m_0
  Inertia Matrix : Constant  Value=eye(3)  VectorParams1D=off
  Inertia Matrix1 : Constant  Value=IB_0  VectorParams1D=off
  MATLAB Function : MATLAB Function  TreatAsAtomicUnit=on  SystemSampleTime=Ts
  MATLAB Function1 : MATLAB Function  TreatAsAtomicUnit=on
  MATLAB Function10 : MATLAB Function  TreatAsAtomicUnit=on  SystemSampleTime=Ts
  MATLAB Function11 : MATLAB Function  TreatAsAtomicUnit=on  SystemSampleTime=Ts
  MATLAB Function12 : MATLAB Function  TreatAsAtomicUnit=on  SystemSampleTime=Ts
  MATLAB Function13 : MATLAB Function  TreatAsAtomicUnit=on  SystemSampleTime=Ts
  MATLAB Function14 : MATLAB Function  TreatAsAtomicUnit=on  SystemSampleTime=Ts
  MATLAB Function15 : MATLAB Function  TreatAsAtomicUnit=on  SystemSampleTime=Ts
  MATLAB Function2 : MATLAB Function  Commented=on  TreatAsAtomicUnit=on  SystemSampleTime=Ts
  MATLAB Function3 : MATLAB Function  TreatAsAtomicUnit=on  SystemSampleTime=Ts
  MATLAB Function4 : MATLAB Function  TreatAsAtomicUnit=on  SystemSampleTime=Ts
  MATLAB Function5 : MATLAB Function  TreatAsAtomicUnit=on  SystemSampleTime=Ts
  MATLAB Function6 : MATLAB Function  TreatAsAtomicUnit=on
  MATLAB Function7 : MATLAB Function  TreatAsAtomicUnit=on
  MATLAB Function8 : MATLAB Function  TreatAsAtomicUnit=on  SystemSampleTime=Ts
  MATLAB Function9 : MATLAB Function  TreatAsAtomicUnit=on  SystemSampleTime=Ts
  Mux : Mux  Inputs=3
  Mux1 : Mux  Inputs=3
  Mux2 : Mux  Inputs=2
  Product : Product  Commented=on  Multiplication=Matrix(*)
  Product7 : Product  Multiplication=Matrix(*)
  Product8 : Product  Multiplication=Matrix(*)
  Scope{,1..17} (18 alike) : Scope
  Sum : Sum  Inputs=|++
  Sum1 : Sum  Inputs=|+-
  Sum2 : Sum  Inputs=|+-
  Sum3 : Sum  Inputs=|-+
  Sum4 : Sum  Inputs=|++
  Sum5 : Sum  Inputs=|-+
  Sum6 : Sum  Inputs=++|
  Sum7 : Sum  Inputs=|-+
  Sum8 : Sum  Inputs=|++
  Vector Concatenate : Concatenate  Mode=Multidimensional array
  Zero-Order Hold2 : ZeroOrderHold  SampleTime=Ts
  Zero-Order Hold3 : ZeroOrderHold  SampleTime=Ts
  Zero-Order Hold5 : ZeroOrderHold  SampleTime=Ts
  u : Outport
  wires:
  "p_d, p_dot_d, p_dotdot_d"/1 -> Zero-Order Hold2/1
  Demux/3 -> MATLAB Function/3(p_dotdot_d)  "p_dotdot_d"
  H/1 -> Vector Concatenate/2  "F2"
  "omega_d, omega_dot_d"/1 -> Zero-Order Hold5/1
  Demux/1 -> Sum1/2  "p_d"
  Demux/2 -> Sum2/2  "p_dot_d"
  F/1 -> Vector Concatenate/1  "F1"
  Sum1/1 -> Gain/1  "z1"
  Sum2/1 -> MATLAB Function/2(z2), Sum/2  "z2"
  Gain/1 -> Sum/1
  Sum/1 -> Scope/1, Sum5/2, Scope17/1, MATLAB Function12/1(s_0), MATLAB Function/1(s)  "s"
  Constant/1 -> MATLAB Function/4(g)
  Constant1/1 -> MATLAB Function/5(lambda)
  Constant2/1 -> MATLAB Function12/2(eta), MATLAB Function/6(eta)
  R_BtoI/1 -> MATLAB Function6/1(R_m), MATLAB Function7/1(R)
  Vector Concatenate/1 -> Product8/2
  MATLAB Function6/1(JR) -> Product8/1
  Inertia Matrix/1 -> MATLAB Function6/2(I_B)
  Product7/1 -> u/1
  Mux2/1 -> Product7/2
  Product8/1 -> MATLAB Function5/1(J)
  MATLAB Function5/1(J_inv) -> Product7/1
  Sum6/1 -> Mux2/1, Scope1/1
  Demux1/1 -> Sum3/1  "omega_d"
  Inertia Matrix1/1 -> MATLAB Function11/9(IBB), MATLAB Function15/3(IB), MATLAB Function2/1(I)
  R_d/1 -> Zero-Order Hold3/1
  Demux1/2 -> MATLAB Function11/7(omega_d_dot)  "omega_dot_d"
  Demux4/2 -> Mux1/2
  Demux2/4 -> MATLAB Function3/4(eta)  "eta"
  Demux2/1 -> Mux/1
  Mux1/1 -> MATLAB Function3/1(epsilon_d)  "epsilon_d"
  Demux4/1 -> Mux1/1
  MATLAB Function7/1(q) -> Scope12/1, Demux2/1
  Mux/1 -> MATLAB Function3/3(epsilon)  "epsilon"
  MATLAB Function1/1(q) -> Scope13/1, Demux4/1
  Demux2/2 -> Mux/2
  Demux2/3 -> Mux/3
  Demux4/3 -> Mux1/3
  Demux4/4 -> MATLAB Function3/2(eta_d)  "eta_d"
  MATLAB Function3/1(eta_tilde) -> Scope14/1, MATLAB Function10/2(eta_tilde), MATLAB Function4/1(eta_tilde), MATLAB Function8/1(eta_tilde)
  MATLAB Function8/1(G) -> MATLAB Function15/2(G), MATLAB Function11/4(G), MATLAB Function9/1(G)
  omega_B/1 -> MATLAB Function11/8(omega_B), Sum3/2  "omega_B"
  Sum3/1 -> Scope11/1, MATLAB Function11/6(omega_tilde), MATLAB Function10/3(omega_tilde), MATLAB Function9/2(omega_tilde)  "omega_tilde"
  MATLAB Function9/1(z2) -> Scope10/1, MATLAB Function11/2(z2), Sum4/2
  MATLAB Function4/1(z1) -> Scope9/1, Gain1/1
  Gain1/1 -> Sum4/1
  Constant4/1 -> MATLAB Function14/2(eta), MATLAB Function11/10(eta)
  Constant3/1 -> MATLAB Function11/3(lambda)
  MATLAB Function10/1(G_dot) -> MATLAB Function11/5(G_dot)
  MATLAB Function12/1(int_arg) -> Scope16/1, Discrete-Time Integrator/1
  Discrete-Time Integrator/1 -> Sum5/1
  Sum5/1 -> MATLAB Function13/1(s)  "new s"
  Constant5/1 -> MATLAB Function13/2(M)
  MATLAB Function13/1(u1) -> Sum6/1, Scope3/1
  MATLAB Function/1(u) -> Gain8/1
  Discrete-Time Integrator1/1 -> Scope7/1, Sum7/1
  Constant6/1 -> MATLAB Function15/4(M)
  Sum4/1 -> Scope2/1, Sum7/2, MATLAB Function14/1(s_0), MATLAB Function11/1(s)  "s"
  MATLAB Function14/1(int_arg) -> Scope6/1, Discrete-Time Integrator1/1
  Sum7/1 -> Scope5/1, MATLAB Function15/1(s)  "new s"
  MATLAB Function2/1(I_inv) -> Product/1
  p_I/1 -> Sum1/1
  v_I/1 -> Sum2/1
  Zero-Order Hold2/1 -> Demux/1
  Zero-Order Hold3/1 -> MATLAB Function1/1(R)
  Zero-Order Hold5/1 -> Demux1/1
  MATLAB Function15/1(u1) -> Scope4/1, Sum8/2
  Sum8/1 -> Mux2/2
  MATLAB Function11/1(u) -> Scope8/1, Sum8/1
  MATLAB Function3/2(epsilon_tilde) -> Scope15/1, MATLAB Function10/1(eps_tilde), MATLAB Function4/2(eps_tilde), MATLAB Function8/2(eps_tilde)
  Gain8/1 -> Sum6/2

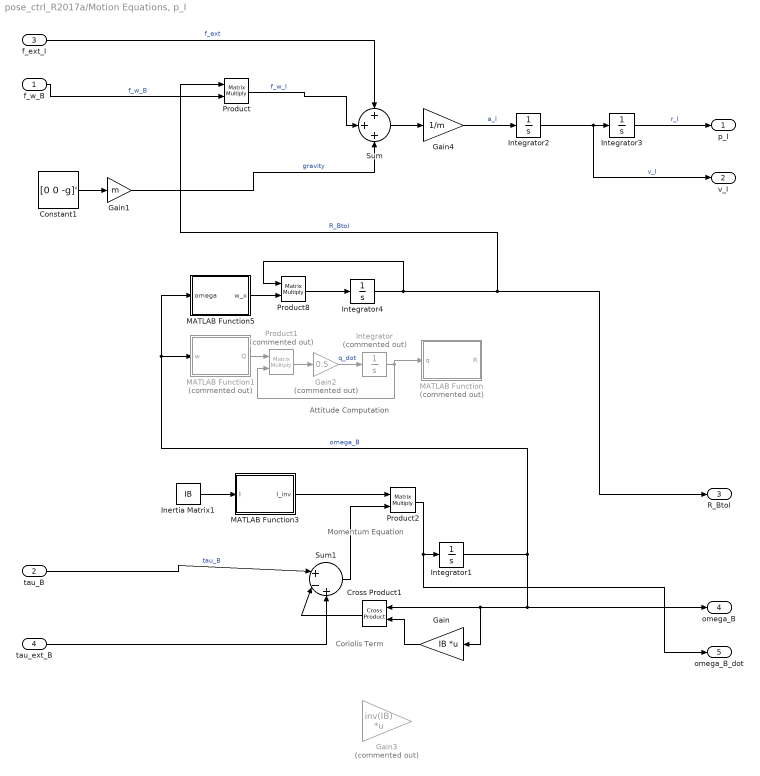
== system pose_ctrl_R2017a/Motion Equations, p_I ==
  note: Momentum Equation
  note: Attitude Computation
  note: Coriolis Term
  "f_w_B " : Inport
  tau_B : Inport  Port=2
  f_ext_I : Inport  Port=3
  tau_ext_B : Inport  Port=4
  Constant1 : Constant  Value=[0 0 -g]'  VectorParams1D=off
  Cross Product1 : vrlib/Utilities/Cross Product
      settings: SourceProductBaseCode=VR
  Gain : Gain  Gain=IB  Multiplication=Matrix(K*u)
  Gain1 : Gain  Gain=m
  Gain2 : Gain  Commented=on  Gain=0.5
  Gain3 : Gain  Commented=on  Gain=inv(IB)  Multiplication=Matrix(K*u)
  Gain4 : Gain  Gain=1/m
  Inertia Matrix1 : Constant  Value=IB  VectorParams1D=off
  Integrator : Integrator  Commented=on  InitialCondition=[0 0 0 1]
  Integrator1 : Integrator  InitialCondition=[0 0 0]'
  Integrator2 : Integrator  InitialCondition=[0;0;0]
  Integrator3 : Integrator  InitialCondition=[0 0 0]'
  Integrator4 : Integrator  InitialCondition=[1 0 0; 0 1 0; 0 0 1]
  MATLAB Function : MATLAB Function  Commented=on  TreatAsAtomicUnit=on
  MATLAB Function1 : MATLAB Function  Commented=on  TreatAsAtomicUnit=on
  MATLAB Function3 : MATLAB Function  TreatAsAtomicUnit=on
  MATLAB Function5 : MATLAB Function  TreatAsAtomicUnit=on
  Product : Product  Multiplication=Matrix(*)
  Product1 : Product  Commented=on  Multiplication=Matrix(*)
  Product2 : Product  Multiplication=Matrix(*)
  Product8 : Product  Multiplication=Matrix(*)
  Sum : Sum  Inputs=+++
  Sum1 : Sum  Inputs=|+-+
  p_I : Outport
  v_I : Outport  Port=2
  R_BtoI : Outport  Port=3
  omega_B : Outport  Port=4
  omega_B_dot : Outport  Port=5
  wires:
  Product2/1 -> omega_B_dot/1, Integrator1/1
  Gain/1 -> Cross Product1/2
  Gain4/1 -> Integrator2/1  "a_I"
  Constant1/1 -> Gain1/1
  Gain2/1 -> Integrator/1  "q_dot"
  Integrator2/1 -> v_I/1, Integrator3/1  "v_I"
  tau_B/1 -> Sum1/1  "tau_B"
  Integrator/1 -> Product1/2, MATLAB Function/1(q)
  Sum1/1 -> Product2/2
  Sum/1 -> Gain4/1
  "f_w_B "/1 -> Product/2  "f_w_B"
  Product1/1 -> Gain2/1
  Gain1/1 -> Sum/3  "gravity"
  Cross Product1/1 -> Sum1/2
  Integrator3/1 -> p_I/1  "r_I"
  MATLAB Function1/1(Q) -> Product1/1
  Integrator1/1 -> omega_B/1, Gain/1, Cross Product1/1, MATLAB Function5/1(omega), MATLAB Function1/1(w)  "omega_B"
  Product/1 -> Sum/2  "f_w_I"
  Product8/1 -> Integrator4/1
  Integrator4/1 -> Product8/1, Product/1, R_BtoI/1  "R_BtoI"
  f_ext_I/1 -> Sum/1  "f_ext"
  tau_ext_B/1 -> Sum1/3
  MATLAB Function3/1(I_inv) -> Product2/1
  Inertia Matrix1/1 -> MATLAB Function3/1(I)
  MATLAB Function5/1(w_x) -> Product8/2

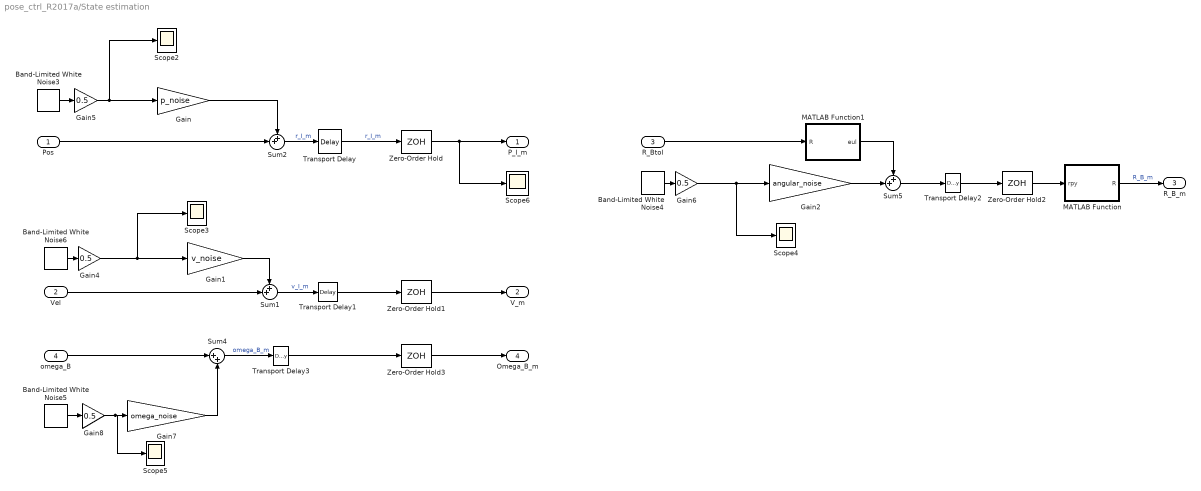
== system pose_ctrl_R2017a/State estimation ==
  Pos : Inport
  Vel : Inport  Port=2
  R_BtoI : Inport  Port=3
  omega_B : Inport  Port=4
  Band-Limited White Noise3 : simulink/Sources/Band-Limited White Noise  Cov=[0.01; 0.01; 0.01]  Ts=Ts  seed=[22352; 29655; 12541]  VectorParams1D=off
  Band-Limited White Noise4 : simulink/Sources/Band-Limited White Noise  Cov=[0.01; 0.01; 0.01]  Ts=Ts  seed=[11351; 22653; 52546]  VectorParams1D=off
  Band-Limited White Noise5 : simulink/Sources/Band-Limited White Noise  Cov=[0.01; 0.01; 0.01]  Ts=Ts  seed=[12451; 82653; 82546]  VectorParams1D=off
  Band-Limited White Noise6 : simulink/Sources/Band-Limited White Noise  Cov=[0.01; 0.01; 0.01]  Ts=Ts  seed=[22351; 29653; 12546]  VectorParams1D=off
  Gain : Gain  Gain=p_noise
  Gain1 : Gain  Gain=v_noise
  Gain2 : Gain  Gain=angular_noise
  Gain{4..6,8} (4 alike) : Gain  Gain=0.5
  Gain7 : Gain  Gain=omega_noise
  MATLAB Function : MATLAB Function  TreatAsAtomicUnit=on
  MATLAB Function1 : MATLAB Function  TreatAsAtomicUnit=on
  Scope{2..6} (5 alike) : Scope
  Sum1 : Sum  Inputs=++|
  Sum2 : Sum  Inputs=++|
  Sum4 : Sum  Inputs=|++
  Sum5 : Sum  Inputs=++|
  Transport Delay{,1..3} (4 alike) : TransportDelay  DelayTime=T_delay  InitialOutput=[0;0;0]
  Zero-Order Hold{,1..3} (4 alike) : ZeroOrderHold  SampleTime=Ts
  P_I_m : Outport
  V_m : Outport  Port=2
  R_B_m : Outport  Port=3
  Omega_B_m : Outport  Port=4
  wires:
  R_BtoI/1 -> MATLAB Function1/1(R)
  Gain1/1 -> Sum1/1
  Band-Limited White Noise6/1 -> Gain4/1
  omega_B/1 -> Sum4/1
  Sum2/1 -> Transport Delay/1  "r_I_m"
  Transport Delay1/1 -> Zero-Order Hold1/1
  Gain2/1 -> Sum5/2
  Transport Delay2/1 -> Zero-Order Hold2/1
  Sum5/1 -> Transport Delay2/1
  Transport Delay3/1 -> Zero-Order Hold3/1
  Gain5/1 -> Scope2/1, Gain/1
  Band-Limited White Noise3/1 -> Gain5/1
  Vel/1 -> Sum1/2
  Zero-Order Hold1/1 -> V_m/1
  Zero-Order Hold3/1 -> Omega_B_m/1
  MATLAB Function/1(R) -> R_B_m/1  "R_B_m"
  MATLAB Function1/1(eul) -> Sum5/1
  Band-Limited White Noise5/1 -> Gain8/1
  Gain7/1 -> Sum4/2
  Sum4/1 -> Transport Delay3/1  "omega_B_m"
  Gain4/1 -> Scope3/1, Gain1/1
  Pos/1 -> Sum2/2
  Transport Delay/1 -> Zero-Order Hold/1  "r_I_m"
  Zero-Order Hold/1 -> P_I_m/1, Scope6/1
  Band-Limited White Noise4/1 -> Gain6/1
  Sum1/1 -> Transport Delay1/1  "v_I_m"
  Gain/1 -> Sum2/1
  Gain8/1 -> Scope5/1, Gain7/1
  Gain6/1 -> Scope4/1, Gain2/1
  Zero-Order Hold2/1 -> MATLAB Function/1(rpy)

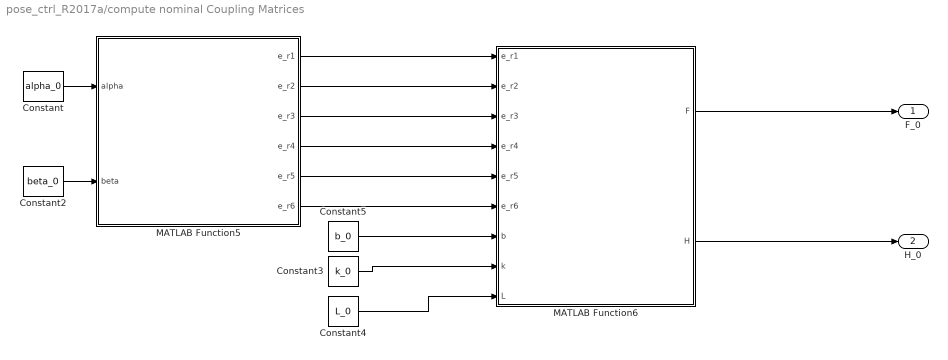
== system pose_ctrl_R2017a/compute nominal Coupling Matrices ==
  Constant : Constant  Value=alpha_0
  Constant2 : Constant  Value=beta_0
  Constant3 : Constant  Value=k_0
  Constant4 : Constant  Value=L_0
  Constant5 : Constant  Value=b_0
  MATLAB Function5 : MATLAB Function  TreatAsAtomicUnit=on
  MATLAB Function6 : MATLAB Function  TreatAsAtomicUnit=on
  F_0 : Outport
  "H_0 " : Outport  Port=2
  wires:
  MATLAB Function6/1(F) -> F_0/1
  MATLAB Function6/2(H) -> "H_0 "/1
  Constant5/1 -> MATLAB Function6/7(b)
  Constant/1 -> MATLAB Function5/1(alpha)
  Constant2/1 -> MATLAB Function5/2(beta)
  Constant3/1 -> MATLAB Function6/8(k)
  MATLAB Function5/5(e_r5) -> MATLAB Function6/5(e_r5)
  MATLAB Function5/1(e_r1) -> MATLAB Function6/1(e_r1)
  MATLAB Function5/4(e_r4) -> MATLAB Function6/4(e_r4)
  MATLAB Function5/3(e_r3) -> MATLAB Function6/3(e_r3)
  MATLAB Function5/2(e_r2) -> MATLAB Function6/2(e_r2)
  Constant4/1 -> MATLAB Function6/9(L)
  MATLAB Function5/6(e_r6) -> MATLAB Function6/6(e_r6)

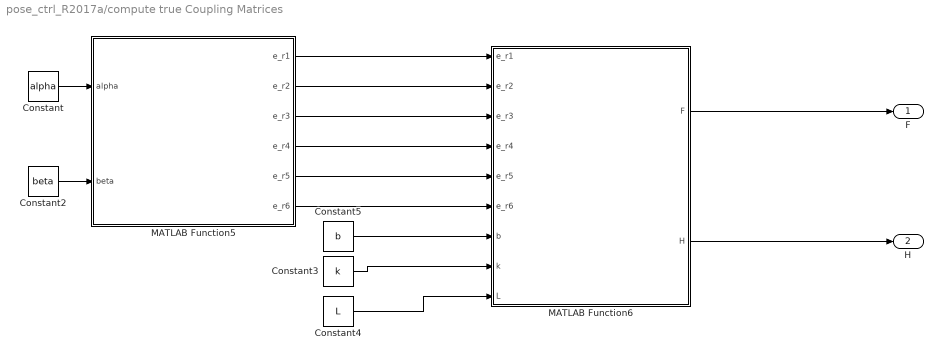
== system pose_ctrl_R2017a/compute true Coupling Matrices ==
  Constant : Constant  Value=alpha
  Constant2 : Constant  Value=beta
  Constant3 : Constant  Value=k
  Constant4 : Constant  Value=L
  Constant5 : Constant  Value=b
  MATLAB Function5 : MATLAB Function  TreatAsAtomicUnit=on
  MATLAB Function6 : MATLAB Function  TreatAsAtomicUnit=on
  F : Outport
  H : Outport  Port=2
  wires:
  MATLAB Function5/6(e_r6) -> MATLAB Function6/6(e_r6)
  Constant4/1 -> MATLAB Function6/9(L)
  MATLAB Function5/2(e_r2) -> MATLAB Function6/2(e_r2)
  MATLAB Function5/3(e_r3) -> MATLAB Function6/3(e_r3)
  MATLAB Function5/4(e_r4) -> MATLAB Function6/4(e_r4)
  MATLAB Function5/1(e_r1) -> MATLAB Function6/1(e_r1)
  MATLAB Function5/5(e_r5) -> MATLAB Function6/5(e_r5)
  Constant3/1 -> MATLAB Function6/8(k)
  Constant2/1 -> MATLAB Function5/2(beta)
  Constant/1 -> MATLAB Function5/1(alpha)
  Constant5/1 -> MATLAB Function6/7(b)
  MATLAB Function6/2(H) -> H/1
  MATLAB Function6/1(F) -> F/1

== matlab function pose_ctrl_R2017a/Motion Equations, p_I/MATLAB Function ==
  data: q input; R output
function R = Quat2R(q)
% compute R from quaternion input

R = [q(1)^2 - q(2)^2 - q(3)^2 + q(4)^2,  2*(q(1)*q(2) - q(3)*q(4)),          2*(q(1)*q(3) + q(2)*q(4));
     2*(q(1)*q(2) + q(3)*q(4)),         -q(1)^2 + q(2)^2 - q(3)^2 + q(4)^2,  2*(q(2)*q(3) - q(1)*q(4));
     2*(q(1)*q(3) - q(2)*q(4)),          2*(q(2)*q(3) + q(1)*q(4)),         -q(1)^2 - q(2)^2 + q(3)^2 + q(4)^2];

== matlab function pose_ctrl_R2017a/Motion Equations, p_I/MATLAB Function1 ==
  data: w input; Q output
function Q = omegaSkew(w)
%#codegen

Q = [0 w(3) -w(2) w(1);
    -w(3) 0 w(1) w(2);
    w(2) -w(1) 0 w(3);
    -w(1) -w(2) -w(3) 0];

== matlab function pose_ctrl_R2017a/Motion Equations, p_I/MATLAB Function5 ==
  data: omega input; w_x output
function w_x = omegaSkew3D(omega)

w_x = [0 -omega(3) omega(2);
        omega(3) 0 -omega(1);
        -omega(2) omega(1) 0];

== matlab function pose_ctrl_R2017a/Feedback Linearization Control [Raj15]/MATLAB Function ==
  data: J input; J_inv output
function J_inv = inverse(J)

J_inv = inv(J);

== matlab function pose_ctrl_R2017a/MATLAB Function4 ==
  data: R input; eul output
function eul = DCM2Euler(R)

%Roll
phi = atan2d(R(3,2),R(3,3));

%Pitch
psi = atan2d(-R(3,1),sqrt(R(1,1)^2 + R(2,1)^2));

%Yaw
gamma = atan2d(R(2,1),R(1,1));

eul=[phi;psi;gamma];

== matlab function pose_ctrl_R2017a/compute true Coupling Matrices/MATLAB Function5 ==
  data: e_r1 output; e_r2 output; e_r3 output; e_r4 output; e_r5 output; e_r6 output; alpha input; beta input
function [e_r1, e_r2, e_r3, e_r4, e_r5, e_r6] = computeThrustDirections(alpha, beta)

e_r = zeros(3,6);
for it = 1:6
    alpha_i = alpha(it);
    beta_i = beta(it);
    gamma_i = (it-1)*pi/3 - pi/6;
    ca = cos(alpha_i);
    sa = sin(alpha_i);
    cb = cos(beta_i);
    sb = sin(beta_i);
    cy = cos(gamma_i);
    sy = sin(gamma_i);
    
    e_r(:,it) = [ca*sb*cy + sa*sy;
                ca*sb*sy - sa*cy;
                ca*cb];
            
end

e_r1 = e_r(:,1);
e_r2 = e_r(:,2);
e_r3 = e_r(:,3);
e_r4 = e_r(:,4);
e_r5 = e_r(:,5);
e_r6 = e_r(:,6);

== matlab function pose_ctrl_R2017a/compute true Coupling Matrices/MATLAB Function6 ==
  data: F output; e_r1 input; e_r2 input; e_r3 input; e_r4 input; e_r5 input; e_r6 input; b input; k input; L input; H output
function [F,H]= computeCouplingMatrix(e_r1, e_r2, e_r3, e_r4, e_r5, e_r6, b, k, L)
% u = w^2

F = zeros(3,6);
H = zeros(3,6);

e_r = [e_r1 e_r2 e_r3 e_r4 e_r5 e_r6];

for it = 1:6
    gamma_i = (it-1)*pi/3;
   
    % thrust direction
    e_ri = e_r(:,it);
    
    % rotor position vector
    r_Ti =  L * [cos(gamma_i);
            sin(gamma_i);
            0];
        
    % Thrust force
    F(:,it) = k*e_ri;   
    
    % thrust and drag moment
    H(:,it) = k * cross(r_Ti, e_ri) + b * (-1)^it * e_ri;
    

    
end

== matlab function pose_ctrl_R2017a/Feedback Linearization Control [Raj15]/MATLAB Function1 ==
  data: R_m input; JR output; I_B input
function JR = computeJR(R_m, I_B)
JR = [R_m zeros(3);
     zeros(3) inv(I_B) ];

== matlab function pose_ctrl_R2017a/Trajectory Generator ==
  data: t input; p_d output; p_d_dot output; p_d_dotdot output; R_d output; omega_d output; omega_d_dot output; T_D output; T_D_dot output
function [p_d, p_d_dot, p_d_dotdot, R_d, omega_d, omega_d_dot, T_D, T_D_dot] = createTrajectory(t)

if t < 10
    %zeros
    % 
    p_d = [0;0;0];
    p_d_dot = [0;0;0];
    p_d_dotdot = [0;0;0];
    R_d = eye(3);
    omega_d = [0;0;0];
    omega_d_dot = [0;0;0];
    T_D = zeros(6,1);
    T_D_dot = zeros(6,1);

else
    p_d = [1;0.75;0];
    p_d_dot = [0;0;0];
    p_d_dotdot = [0;0;0];
    
    ct = cosd(7.5);
    st = sind(7.5);
    ct2 = cosd(10);
    st2 = sind(10);
    R_d = [ct, 0, st; 
            0, 1, 0;
            -st, 0, ct]*[1 0 0;
            0 ct2, -st2; 
           0 st2, ct2];
    omega_d = [0;0;0];
    omega_d_dot = [0;0;0];
    T_D = zeros(6,1);
    T_D_dot = zeros(6,1);
    
%     
%         t = t-10;
%     xa = 0;
%     xe = 1;
%     te = 5;
%     x = xa + 10*(xe-xa)*t^3/te^3 - 15*(xe-xa)*t^4/te^4 + 6*(xe-xa)*t^5/te^5;
%     x_dot = 3*10*(xe-xa)*t^2/te^3 - 4*15*(xe-xa)*t^3/te^4 + 5*6*(xe-xa)*t^4/te^5;
%     x_dot_dot = 6*10*(xe-xa)*t/te^3 - 12*15*(xe-xa)*t^2/te^4 + 20*6*(xe-xa)*t^3/te^5;
%     if (t> te)
%         x = xe;
%         x_dot = 0;
%         x_dot_dot = 0;
%     end
%     p_d = [x;0;x];
%     p_d_dot = [x_dot;0;x_dot];
%     p_d_dotdot = [x_dot_dot;0;x_dot_dot];
%     
%     xe = 0.5;
%     x = xa + 10*(xe-xa)*t^3/te^3 - 15*(xe-xa)*t^4/te^4 + 6*(xe-xa)*t^5/te^5;
%     x_dot = 3*10*(xe-xa)*t^2/te^3 - 4*15*(xe-xa)*t^3/te^4 + 5*6*(xe-xa)*t^4/te^5;
%     x_dot_dot = 6*10*(xe-xa)*t/te^3 - 12*15*(xe-xa)*t^2/te^4 + 20*6*(xe-xa)*t^3/te^5;
%     if (t> te)
%         x = xe;
%         x_dot = 0;
%         x_dot_dot = 0;
%     end
%     p_d(3) = x;
%     p_d_dot(3) = x_dot;
%     p_d_dotdot(3) = x_dot_dot;
%     
%     a = 2*pi/te;
%     ct = cos(a*t);
%     st = sin(a*t);
%     
%     R_d = [ct, -st, 0; 
%            st, ct, 0;
%            0 0 1];
%     R_d_dot = [-a*st, -a*ct, 0;
%                 a*ct, -a*st, 0;
%                 0 0 0];
%     R_d_dotdot = [-a*a*ct, a*a*st, 0;
%                    -a*a*st, -a*a*ct, 0;
%                    0 0 0];
%                
%     T_d_tilde = [R_d', -R_d'*p_d; 0,0,0,1]*[R_d_dot p_d_dot; 0,0,0,0];
%     
%     omega_d = skew2vec(T_d_tilde(1:3,1:3));
%     
%     T_d_tilde_dot = [R_d_dot'*R_d_dot+R_d'*R_d_dotdot, R_d_dot'*p_d_dot+R_d'*p_d_dotdot;
%         0,0,0,0];
%     
%     omega_d_dot = skew2vec(T_d_tilde_dot(1:3,1:3));
%     
%     T_D = [omega_d; T_d_tilde(1:3,4)];
%     T_D_dot = [omega_d_dot; T_d_tilde_dot(1:3,4)];
%     
%     if t>te
%         R_d = eye(3);
%         omega_d = [0;0;0];
%         omega_d_dot = [0;0;0];
%         T_D = zeros(6,1);
%         T_D_dot = zeros(6,1);
%     end
end
% 
% p_d = [0;0;0];
%     p_d_dot = [0;0;0];
%     p_d_dotdot = [0;0;0];
%     R_d = eye(3);
%     omega_d = [0;0;0];
%     omega_d_dot = [0;0;0];
%     T_D = zeros(6,1);
%     T_D_dot = zeros(6,1);

== matlab function pose_ctrl_R2017a/DC Motor Dynamics /MATLAB Function2 ==
  data: u input; y output
function y = fcn(u)

y = sqrt(abs(u))*sign(u);

== matlab function pose_ctrl_R2017a/DC Motor Dynamics /MATLAB Function3 ==
  data: u input; y output
function y = fcn(u)

y = u^2*sign(u);

== matlab function pose_ctrl_R2017a/Feedback Linearization Control [Raj15]/MATLAB Function3 ==
  data: u input; y output
function y = transpose(u)

y = u';

== matlab function pose_ctrl_R2017a/Feedback Linearization Control [Raj15]/MATLAB Function5 ==
  data: R_d input; e_R output; R_BtoI input
function e_R = compute_e_R(R_d, R_BtoI)

A = R_d' * R_BtoI - R_BtoI' * R_d;

e_R = 0.5 * [A(3,2); A(1,3); A(2,1)];

== matlab function pose_ctrl_R2017a/Integral Backstepping/MATLAB Function1 ==
  data: R input; q output
function q   = DCM2Quat(R)

%%%%%%%%%%%%%%%%%%%%%%%%%%%%%%%%%%%%%%%%%%%%%%%%%%%%%%%%%%%%%%%%%%%%%%%%%%%
%
% M-file: Tool_DCM2Quat
%         -> impelmeted as M-Function
% Author: Marcel Tkocz
% Version: 27.01.2008
%
% Description:
%   This Function converts roll-pitch-yaw angels into their quaternion
%   equivalents.
%
% Inputs:
%   Orientation ... orientation in roll-pitch-yaw angels
%
% Outputs:
%   q           ... orientation in quaternions
%   
%%%%%%%%%%%%%%%%%%%%%%%%%%%%%%%%%%%%%%%%%%%%%%%%%%%%%%%%%%%%%%%%%%%%%%%%%%%

%--------------------------------------------------------------------------
% Calculation of Quaternions based on q1
%--------------------------------------------------------------------------
q = [0 0 0 1]';

if (1 + R(1,1) - R(2,2) - R(3,3)) > 0 
    q1 = 1/2*sqrt(1 + R(1,1) - R(2,2) - R(3,3));
    q2 = 1/(4*q1)*( R(1,2) + R(2,1));
    q3 = 1/(4*q1)*( R(1,3) + R(3,1));
    q4 = 1/(4*q1)*(-R(2,3) + R(3,2));

    if round(q1) ~= 0
        q = [q1; q2; q3; q4];
    end
end

%--------------------------------------------------------------------------
% Calculation of Quaternions based on q2
%--------------------------------------------------------------------------

if (1 - R(1,1) + R(2,2) - R(3,3)) > 0
    q2 = 1/2*sqrt(1 - R(1,1) + R(2,2) - R(3,3));
    q1 = 1/(4*q2)*( R(1,2) + R(2,1));
    q3 = 1/(4*q2)*( R(2,3) + R(3,2));
    q4 = 1/(4*q2)*( R(1,3) - R(3,1));

    if round(q2) ~= 0
        q = [q1; q2; q3; q4];
    end
end

%--------------------------------------------------------------------------
% Calculation of Quaternions based on q3
%--------------------------------------------------------------------------

if (1 - R(1,1) - R(2,2) + R(3,3)) > 0
    q3 = 1/2*sqrt(1 - R(1,1) - R(2,2) + R(3,3));
    q1 = 1/(4*q3)*( R(1,3) + R(3,1));
    q2 = 1/(4*q3)*( R(2,3) + R(3,2));
    q4 = 1/(4*q3)*(-R(1,2) + R(2,1));

    if round(q3) ~= 0
        q = [q1; q2; q3; q4];
    end
end

%--------------------------------------------------------------------------
% Calculation of Quaternions based on q4
%--------------------------------------------------------------------------

if (1 + R(1,1) + R(2,2) + R(3,3)) > 0
    q4 = 1/2*sqrt(1 + R(1,1) + R(2,2) + R(3,3));
    q1 = 1/(4*q4)*(-R(2,3) + R(3,2));
    q2 = 1/(4*q4)*(-R(3,1) + R(1,3));
    q3 = 1/(4*q4)*(-R(1,2) + R(2,1));

    if round(q4) ~= 0
        q = [q1; q2; q3; q4];
    end
end


end

== matlab function pose_ctrl_R2017a/Integral Backstepping/MATLAB Function ==
  data: epsilon_d input; eta_d input; epsilon input; eta input; eta_tilde output; epsilon_tilde output; epsilon_tilde_T output; skew_eps_tilde output
function [eta_tilde, epsilon_tilde, epsilon_tilde_T, skew_eps_tilde] = calc_q_tilde(epsilon_d, eta_d, epsilon, eta)

eta_tilde = eta_d*eta + epsilon_d'*epsilon;

epsilon_tilde = eta_d * epsilon - eta*epsilon_d - vec2skew(epsilon_d)*epsilon;

epsilon_tilde_T = epsilon_tilde';

skew_eps_tilde = vec2skew(epsilon_tilde);

== matlab function pose_ctrl_R2017a/Integral Backstepping/MATLAB Function2 ==
  data: eta_tilde input; z1 output; eps_tilde input
function z1 = compute_z1(eta_tilde, eps_tilde)

z1 = [1-abs(eta_tilde);
    eps_tilde];

== matlab function pose_ctrl_R2017a/Integral Backstepping/MATLAB Function3 ==
  data: eta_tilde input; G output; eps_tilde input
function G = compute_G(eta_tilde, eps_tilde)

if (eta_tilde >= 0)
    sig = 1;
else
    sig = -1;
end

G = [sig*eps_tilde';
    eye(3)*eta_tilde + vec2skew(eps_tilde)]';

== matlab function pose_ctrl_R2017a/Integral Backstepping/MATLAB Function4 ==
  data: K1 input; alpha_dot output; G input; z1 input; z2 input; omega_tilde input; eta_tilde input; eps_tilde input; K3 input; Xsi input
function alpha_dot  = compute_alpha_dot(K1,G,z1,z2, omega_tilde, eta_tilde, eps_tilde, K3, Xsi)

eta_dot = -0.5*eps_tilde'*omega_tilde;

eps_dot = 0.5*(eta_tilde*eye(3) + vec2skew(eps_tilde))*omega_tilde;

if eta_tilde >= 0
    sig = 1;
else
    sig = -1;
end

G_dot = [sig*eps_dot';
        eta_dot*eye(3) + vec2skew(eps_dot)]';

% alpha_dot = -K1 ( G_dot * z1 + G * z1_dot) 
% - 2 (-inv(GT)G_dot inv(GT) * K3 * Xsi + inv(GT)K3*z1
%alpha_dot1 = -K1*(G_dot*z1  + G*(-0.5*G'*K1*G*z1 + 0.5*G'*z2));
alpha_dot1 = -K1*(G_dot*z1  + G*(0.5*G.'*omega_tilde));

%alpha_dot2 = -2*(-pGT*(G_dot.')*pGT*K3*Xsi + pGT*K3*z1);
alpha_dot2 = -2*(G_dot*K3*Xsi + G*K3*z1);
alpha_dot=alpha_dot1+ alpha_dot2;

== matlab function pose_ctrl_R2017a/Integral Backstepping/MATLAB Function5 ==
  data: J input; J_inv output
function J_inv = inverse(J)

J_inv = inv(J);

== matlab function pose_ctrl_R2017a/Integral Backstepping/MATLAB Function6 ==
  data: R_m input; JR output; I_B input
function JR = computeJR(R_m, I_B)
JR = [R_m zeros(3);
     zeros(3) inv(I_B) ];
